simulink model "extended_discrete_kalman_filter"  (R2015b)
settings: Solver=VariableStepAuto  StartTime=0.0  StopTime=10.0  RelTol=1e-3
settings Model: Creator=mgreiff  LastModifiedBy=mgreiff

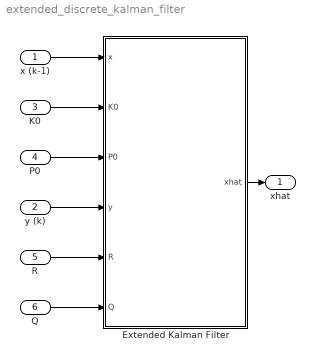
== system extended_discrete_kalman_filter ==
  x (k-1) : Inport
  y (k) : Inport  Port=2
  K0 : Inport  Port=3
  P0 : Inport  Port=4
  R : Inport  Port=5
  Q : Inport  Port=6
  Extended Kalman Filter : MATLAB Function  TreatAsAtomicUnit=on
  xhat : Outport
  wires:
  Extended Kalman Filter/1(xhat) -> xhat/1
  x (k-1)/1 -> Extended Kalman Filter/1(x)
  y (k)/1 -> Extended Kalman Filter/4(y)
  K0/1 -> Extended Kalman Filter/2(K0)
  P0/1 -> Extended Kalman Filter/3(P0)
  R/1 -> Extended Kalman Filter/5(R)
  Q/1 -> Extended Kalman Filter/6(Q)

== matlab function extended_discrete_kalman_filter/Extended Kalman Filter ==
  data: x input; K0 input; P0 input; y input; xhat output; R input; Q input
function xhat = fcn(x, K0, P0, y, R, Q)
%#codegen
persistent P K

if isempty(P)
    P = P0;
    K = K0;
end

%% Predictor step
% Approximate Jacobian at the previous step
J = 1;  % Evaluate jacobian around x
%xf = x; % Evaluate next state in the discrete formulation
%yf = x; % Evaluate next y in the discrete formulation
Pf = J * P * J' + Q;

xf = 1;
yf = 1;
y = 1;

%% Corrector step
xa = xf + K * (y - yf);
Jh = 1; % Evaluate jacobian around xf
K = Pf * J / (J * P * J' + R);
P = (eye(1) - K * Jh) * Pf;
xhat = xa;
